simulink library "Lidar_WindReconstruction_16b"  (Simulink 8.8)
settings: Solver=VariableStepAuto  StartTime=0.0  StopTime=10.0  RelTol=1e-3
undefined symbols (not defined in the file): Atmosphere, CRM, LIDAR, SimConfig, WindReconstruction
libraries: simulink x1
settings Model: Creator=cava_da  LastModifiedBy=cava_da

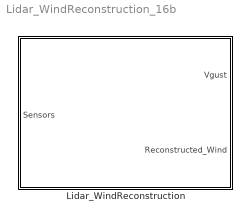
== system Lidar_WindReconstruction_16b ==
  Lidar_WindReconstruction : Subsystem

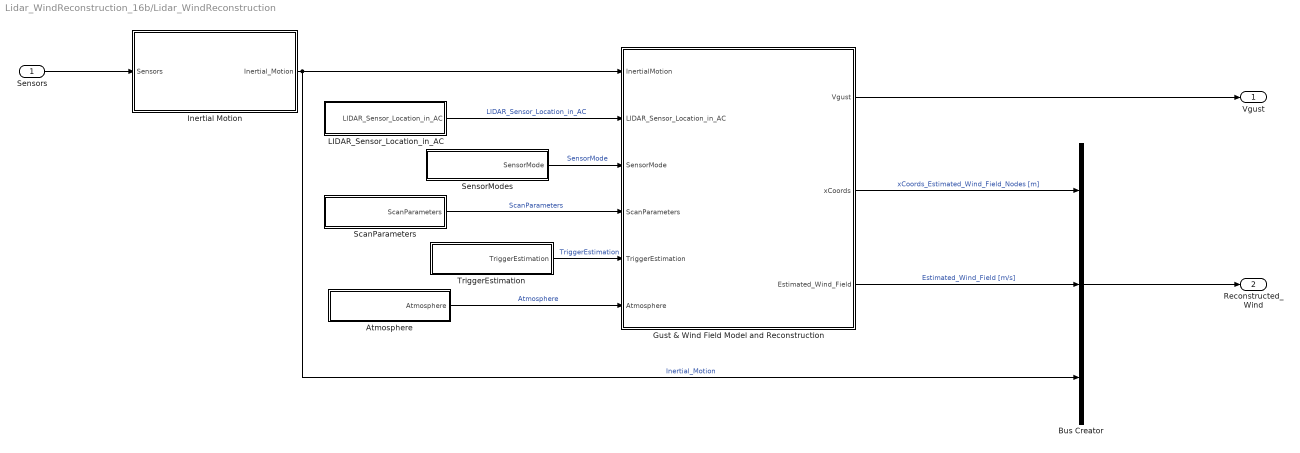
== system Lidar_WindReconstruction_16b/Lidar_WindReconstruction ==
  Sensors : Inport
  Atmosphere : Subsystem
  Bus Creator : BusCreator  Inputs=3
  Gust & Wind Field Model and Reconstruction : Subsystem
  Inertial Motion : Subsystem
  LIDAR_Sensor_Location_in_AC : Subsystem
  ScanParameters : Subsystem
  SensorModes : Subsystem
  TriggerEstimation : Subsystem
  Vgust : Outport
  Reconstructed_Wind : Outport  Port=2
  wires:
  Sensors/1 -> Inertial Motion/1(Sensors)
  LIDAR_Sensor_Location_in_AC/1(LIDAR_Sensor_Location_in_AC) -> Gust & Wind Field Model and Reconstruction/2(LIDAR_Sensor_Location_in_AC)  "LIDAR_Sensor_Location_in_AC"
  SensorModes/1(SensorMode) -> Gust & Wind Field Model and Reconstruction/3(SensorMode)  "SensorMode"
  ScanParameters/1(ScanParameters) -> Gust & Wind Field Model and Reconstruction/4(ScanParameters)  "ScanParameters"
  TriggerEstimation/1(TriggerEstimation) -> Gust & Wind Field Model and Reconstruction/5(TriggerEstimation)  "TriggerEstimation"
  Inertial Motion/1(Inertial_Motion) -> Bus Creator/3, Gust & Wind Field Model and Reconstruction/1(InertialMotion)  "Inertial_Motion"
  Gust & Wind Field Model and Reconstruction/2(xCoords) -> Bus Creator/1  "xCoords_Estimated_Wind_Field_Nodes [m]"
  Gust & Wind Field Model and Reconstruction/3(Estimated_Wind_Field) -> Bus Creator/2  "Estimated_Wind_Field [m/s]"
  Gust & Wind Field Model and Reconstruction/1(Vgust) -> Vgust/1
  Atmosphere/1(Atmosphere) -> Gust & Wind Field Model and Reconstruction/6(Atmosphere)  "Atmosphere"
  Bus Creator/1 -> Reconstructed_Wind/1

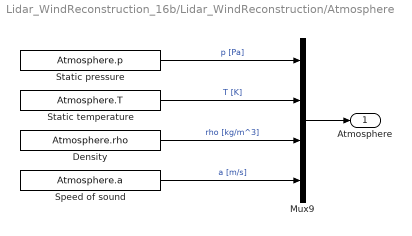
== system Lidar_WindReconstruction_16b/Lidar_WindReconstruction/Atmosphere ==
  Density : Constant  Value=Atmosphere.rho
  Mux9 : Mux
  Speed of sound : Constant  Value=Atmosphere.a
  Static pressure : Constant  Value=Atmosphere.p
  Static temperature : Constant  Value=Atmosphere.T
  Atmosphere : Outport
  wires:
  Mux9/1 -> Atmosphere/1
  Static pressure/1 -> Mux9/1  "p [Pa]"
  Static temperature/1 -> Mux9/2  "T [K]"
  Density/1 -> Mux9/3  "rho [kg/m^3]"
  Speed of sound/1 -> Mux9/4  "a [m/s]"

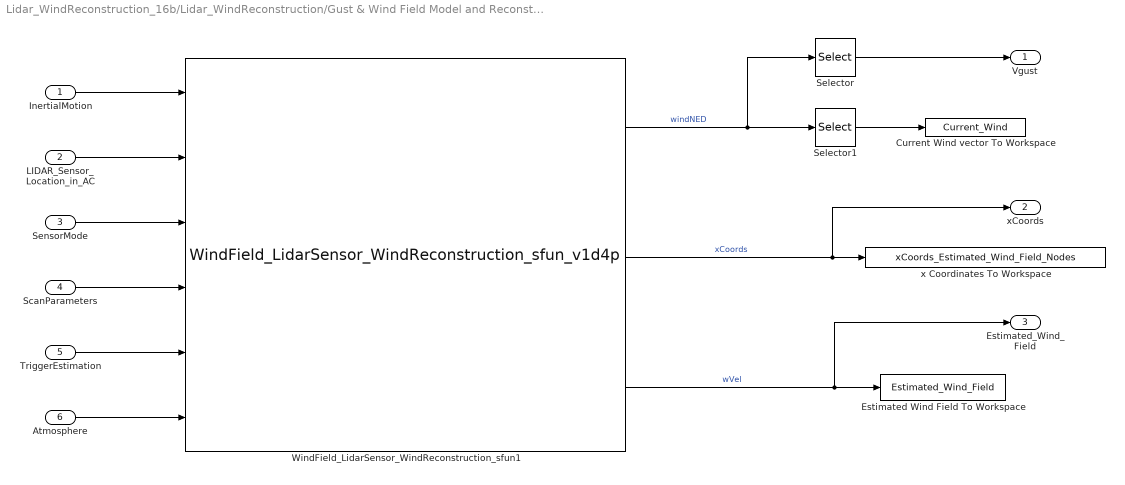
== system Lidar_WindReconstruction_16b/Lidar_WindReconstruction/Gust & Wind Field Model and Reconstruction ==
  InertialMotion : Inport
  LIDAR_Sensor_Location_in_AC : Inport  Port=2
  SensorMode : Inport  Port=3
  ScanParameters : Inport  Port=4
  TriggerEstimation : Inport  Port=5
  Atmosphere : Inport  Port=6
  Current Wind vector To Workspace : ToWorkspace  VariableName=Current_Wind  SaveFormat=Structure  SampleTime=-1
  Estimated Wind Field To Workspace : ToWorkspace  VariableName=Estimated_Wind_Field  SaveFormat=Structure With Time  SampleTime=0.1
      settings: Decimation=SimConfig.Logging.DecimationFactor
  Selector : Selector  IndexOptions=Index vector (dialog)  Indices=3  OutputSizes=1
  Selector1 : Selector  IndexOptions=Index vector (dialog)  Indices=1:3  OutputSizes=1
  WindField_LidarSensor_WindReconstruction_sfun1 : S-Function  FunctionName=WindField_LidarSensor_WindReconstruction_sfun_v1d4p  Parameters=Atmosphere,LIDAR,WindReconstruction  SFunctionDeploymentMode=off  EnableBusSupport=off  mask(Direct detection wind lidar and wind reconstruction (s-function)){}
      mask help:
      | This s-function incorporates the model of a direct detection Doppler wind lidar coupled with a wind reconstruction algorithm based on maximum likelihood estimation. It also serves as the interface between the included wind model and the encompassing aeroelastic aircraft model via the configurable wind output (output port 1).
      | The lidar model and the wind reconstruction algorithm are technically independent modules, but are implemented in the same s-function for performance reasons.
      |
      | Output port 1: wind output, configurable via the parameter Atmosphere.WindConfig
      | Output port 2: x-coordinates of the estimation nodes in geodetic frame and in meters
      | Output port 3: vertical wind speed at the estimation nodes in m/s
      |
      | Output ports 2 and 3 are only updated when a new estimation was triggered via input port 5.
      |
      | Detailed documentation is found under: https://github.com/dlr-ft-gla/GLA-Benchmark/wiki
      |
      |
      |
      | (c) Copyright 2021 DLR e. V.
      |
      | Institute of Flight Systems, 38108 Braunschweig, Germany.
      | Institute of Atmospheric Physics, 82234 Wessling, Germany.
      |
      | Authors:
      | Daniel Kiehn (daniel.kiehn@dlr.de)
      | Nicolas Fezans (nicolas.fezans@dlr.de)
      | Patrick Vrancken (patrick.vrancken@dlr.de)
      |
      | Block and underlying s-function released under CC-BY-ND 4.0 license.
      | https://creativecommons.org/licenses/by-nd/4.0/
      mask Help: For help, please refer to the online documentation of the CRM benchmark model: <a href="matlab: web('https://github.com/dlr-ft-gla/GLA-Benchmark/wiki')">https://github.com/dlr-ft-gla/GLA-Benchmark/wiki</a>.
      mask Display:
      | port_label('input', 1, 'Inertial motion');
      | port_label('input', 2, 'Sensor location in AC');
      | port_label('input', 3, 'Sensor mode');
      | port_label('input', 4, 'Scan parameters');
      | port_label('input', 5, 'Estimation trigger');
      | port_label('input', 6, 'Atmosphere');
      | 
      | port_label('output', 1, 'AC wind inputs');
      | port_label('output', 2, 'x coordinates');
      | port_label('output', 3, 'Estimated wind');
      | 
      | image(imread('DLR_Logo.jpg'),[180,10,81,68])
      | 
      | disp(['DIRECT DETECTION WIND LIDAR\n',...
      | '& WIND RECONSTRUCTION ALGORITHM\n\n\n\n',...
      | '(c) Copyright 2021 DLR e. V.\n\n',...
      | 'Institute of Flight Systems\n',...
      | 'Institute of Atmospheric Physics\n\n',...
      | 'Authors:\n',...
      | 'Daniel Kiehn (daniel.kiehn@dlr.de)\n',...
      | 'Nicolas Fezans (nicolas.fezans@dlr.de)\n',...
      | 'Patrick Vrancken (patrick.vrancken@dlr.de)\n\n\n',...
      | 'Block and underlying s-function\n',...
      | 'released under CC-BY-ND 4.0 license.'])
  x Coordinates To Workspace : ToWorkspace  VariableName=xCoords_Estimated_Wind_Field_Nodes  SaveFormat=Structure With Time  SampleTime=0.1
      settings: Decimation=SimConfig.Logging.DecimationFactor
  Vgust : Outport
  xCoords : Outport  Port=2
  Estimated_Wind_Field : Outport  Port=3
  wires:
  WindField_LidarSensor_WindReconstruction_sfun1/3 -> Estimated_Wind_Field/1, Estimated Wind Field To Workspace/1  "wVel"
  WindField_LidarSensor_WindReconstruction_sfun1/2 -> xCoords/1, x Coordinates To Workspace/1  "xCoords"
  WindField_LidarSensor_WindReconstruction_sfun1/1 -> Selector1/1, Selector/1  "windNED"
  InertialMotion/1 -> WindField_LidarSensor_WindReconstruction_sfun1/1
  LIDAR_Sensor_Location_in_AC/1 -> WindField_LidarSensor_WindReconstruction_sfun1/2
  SensorMode/1 -> WindField_LidarSensor_WindReconstruction_sfun1/3
  ScanParameters/1 -> WindField_LidarSensor_WindReconstruction_sfun1/4
  TriggerEstimation/1 -> WindField_LidarSensor_WindReconstruction_sfun1/5
  Selector/1 -> Vgust/1
  Atmosphere/1 -> WindField_LidarSensor_WindReconstruction_sfun1/6
  Selector1/1 -> Current Wind vector To Workspace/1

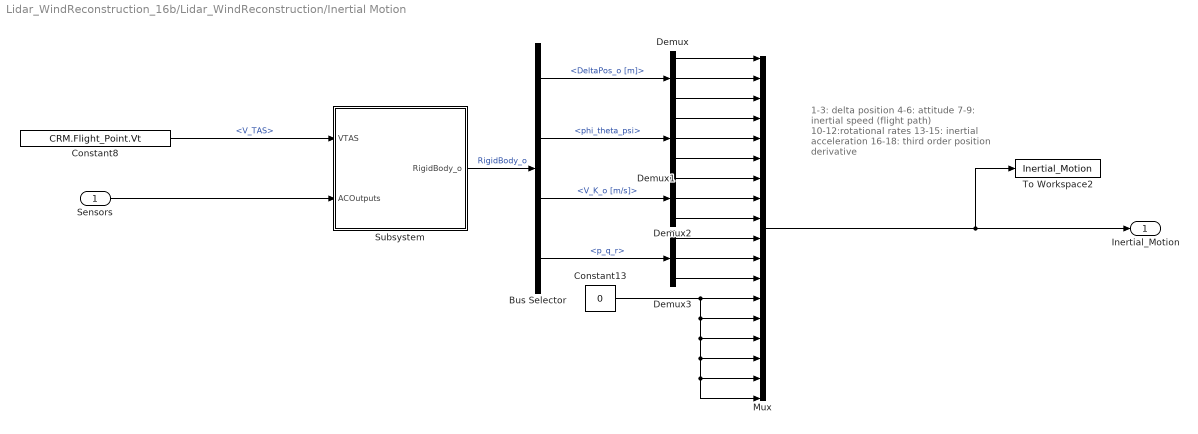
== system Lidar_WindReconstruction_16b/Lidar_WindReconstruction/Inertial Motion ==
  note: 1-3: delta position
      | 4-6: attitude
      | 7-9: inertial speed (flight path)
      | 10-12:rotational rates
      | 13-15: inertial acceleration
      | 16-18: third order position derivative
  Sensors : Inport
  Bus Selector : BusSelector  OutputSignals=DeltaPos_o [m],phi_theta_psi,V_K_o [m/s],p_q_r
  Constant13 : Constant  Value=0
  Constant8 : Constant  Value=CRM.Flight_Point.Vt
  Demux{,1..3} (4 alike) : Demux  Outputs=3
  Mux : Mux  Inputs=18
  Subsystem : Subsystem
  To Workspace2 : ToWorkspace  VariableName=Inertial_Motion  SaveFormat=Structure  SampleTime=-1
      settings: Decimation=SimConfig.Logging.DecimationFactor
  Inertial_Motion : Outport
  wires:
  Bus Selector/4 -> Demux3/1  "<p_q_r>"
  Bus Selector/1 -> Demux/1  "<DeltaPos_o [m]>"
  Bus Selector/2 -> Demux1/1  "<phi_theta_psi>"
  Bus Selector/3 -> Demux2/1  "<V_K_o [m/s]>"
  Demux/1 -> Mux/1
  Demux/2 -> Mux/2
  Demux/3 -> Mux/3
  Demux1/1 -> Mux/4
  Demux1/2 -> Mux/5
  Demux1/3 -> Mux/6
  Demux2/1 -> Mux/7
  Demux2/2 -> Mux/8
  Demux2/3 -> Mux/9
  Demux3/1 -> Mux/10
  Demux3/2 -> Mux/11
  Demux3/3 -> Mux/12
  Sensors/1 -> Subsystem/2(ACOutputs)
  Subsystem/1(RigidBody_o) -> Bus Selector/1  "RigidBody_o"
  Constant8/1 -> Subsystem/1(VTAS)  "<V_TAS>"
  Mux/1 -> Inertial_Motion/1, To Workspace2/1
  Constant13/1 -> Mux/17, Mux/18, Mux/16, Mux/15, Mux/14, Mux/13

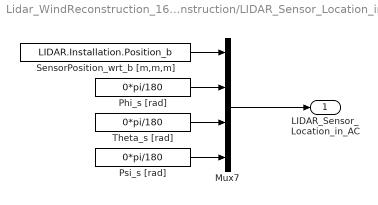
== system Lidar_WindReconstruction_16b/Lidar_WindReconstruction/LIDAR_Sensor_Location_in_AC ==
  Mux7 : Mux
  Phi_s [rad] : Constant  Value=0*pi/180
  Psi_s [rad] : Constant  Value=0*pi/180
  SensorPosition_wrt_b [m,m,m] : Constant  Value=LIDAR.Installation.Position_b
  Theta_s [rad] : Constant  Value=0*pi/180
  LIDAR_Sensor_Location_in_AC : Outport
  wires:
  SensorPosition_wrt_b [m,m,m]/1 -> Mux7/1
  Phi_s [rad]/1 -> Mux7/2
  Theta_s [rad]/1 -> Mux7/3
  Psi_s [rad]/1 -> Mux7/4
  Mux7/1 -> LIDAR_Sensor_Location_in_AC/1

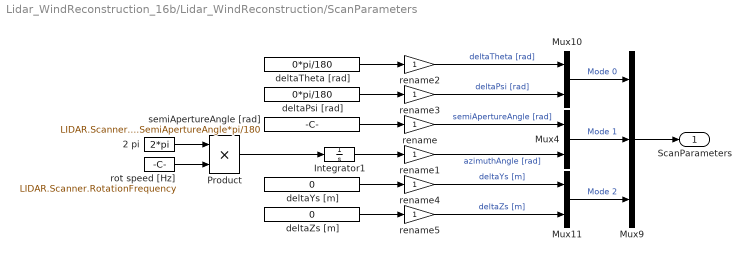
== system Lidar_WindReconstruction_16b/Lidar_WindReconstruction/ScanParameters ==
  2 pi : Constant  Value=2*pi
  Integrator1 : Integrator
  Mux10 : Mux  Inputs=2
  Mux11 : Mux  Inputs=2
  Mux4 : Mux  Inputs=2
  Mux9 : Mux  Inputs=3
  Product : Product  RndMeth=Zero
  deltaPsi [rad] : Constant  Value=0*pi/180  OutDataTypeStr=double
  deltaTheta [rad] : Constant  Value=0*pi/180  OutDataTypeStr=double
  deltaYs [m] : Constant  Value=0  OutDataTypeStr=double
  deltaZs [m] : Constant  Value=0  OutDataTypeStr=double
  rename{,1..5} (6 alike) : Gain
  rot speed [Hz] : Constant  Value=LIDAR.Scanner.RotationFrequency
  semiApertureAngle [rad] : Constant  Value=LIDAR.Scanner.SemiApertureAngle*pi/180  OutDataTypeStr=double
  ScanParameters : Outport
  wires:
  rename3/1 -> Mux10/2  "deltaPsi [rad]"
  rename2/1 -> Mux10/1  "deltaTheta [rad]"
  Mux10/1 -> Mux9/1  "Mode 0"
  rename1/1 -> Mux4/2  "azimuthAngle [rad]"
  rename/1 -> Mux4/1  "semiApertureAngle [rad]"
  rename5/1 -> Mux11/2  "deltaZs [m]"
  rename4/1 -> Mux11/1  "deltaYs [m]"
  Mux4/1 -> Mux9/2  "Mode 1"
  Mux11/1 -> Mux9/3  "Mode 2"
  deltaPsi [rad]/1 -> rename3/1
  deltaTheta [rad]/1 -> rename2/1
  deltaYs [m]/1 -> rename4/1
  deltaZs [m]/1 -> rename5/1
  semiApertureAngle [rad]/1 -> rename/1
  2 pi/1 -> Product/1
  Product/1 -> Integrator1/1
  rot speed [Hz]/1 -> Product/2
  Integrator1/1 -> rename1/1
  Mux9/1 -> ScanParameters/1

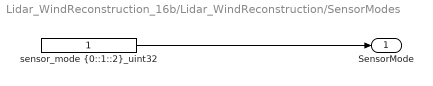
== system Lidar_WindReconstruction_16b/Lidar_WindReconstruction/SensorModes ==
  "sensor_mode {0::1::2}_uint32" : Constant  OutDataTypeStr=uint32
  SensorMode : Outport
  wires:
  "sensor_mode {0::1::2}_uint32"/1 -> SensorMode/1

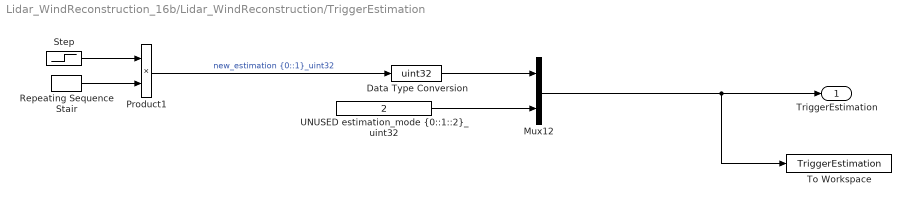
== system Lidar_WindReconstruction_16b/Lidar_WindReconstruction/TriggerEstimation ==
  Data Type Conversion : DataTypeConversion  OutDataTypeStr=uint32
  Mux12 : Mux  Inputs=2
  Product1 : Product  RndMeth=Zero
  Repeating Sequence Stair : simulink/Sources/Repeating Sequence Stair  OutValues=[1 zeros(1,(1/(10*SimConfig.SampleTime))-1)].'  tsamp=-1  OutMin=[]  OutMax=[]  OutDataTypeStr=float('double')  OutputDataTypeScalingMode=Specify via dialog  OutDataType=float('double')  ConRadixGroup=Best Precision: Vector-wise  OutScaling=2^-12
  Step : Step  Time=WindReconstruction.StartEstimationTime  SampleTime=0
  To Workspace : ToWorkspace  VariableName=TriggerEstimation  SaveFormat=Structure  SampleTime=-1
  "UNUSED estimation_mode {0::1::2}_uint32" : Constant  Value=2  OutDataTypeStr=uint32
  TriggerEstimation : Outport
  wires:
  Product1/1 -> Data Type Conversion/1  "new_estimation {0::1}_uint32"
  "UNUSED estimation_mode {0::1::2}_uint32"/1 -> Mux12/2
  Data Type Conversion/1 -> Mux12/1
  Repeating Sequence Stair/1 -> Product1/2
  Step/1 -> Product1/1
  Mux12/1 -> TriggerEstimation/1, To Workspace/1

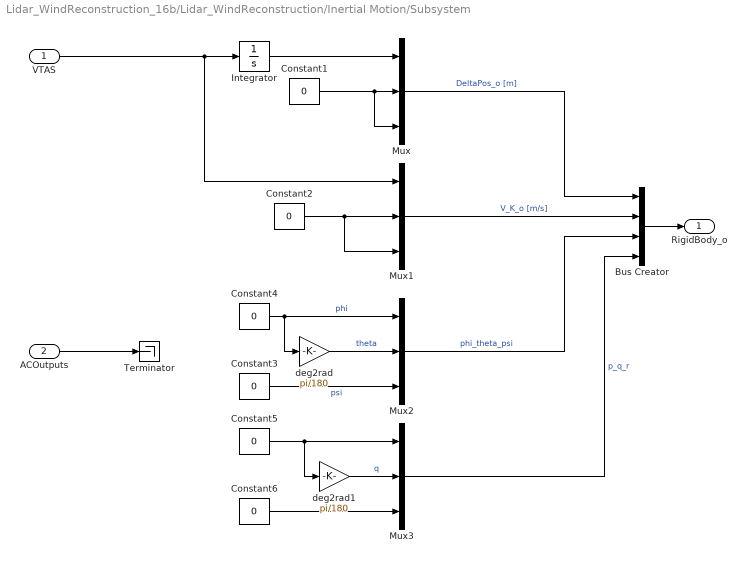
== system Lidar_WindReconstruction_16b/Lidar_WindReconstruction/Inertial Motion/Subsystem ==
  VTAS : Inport
  ACOutputs : Inport  Port=2
  Bus Creator : BusCreator  Inputs=4
  Constant{1..6} (6 alike) : Constant  Value=0
  Integrator : Integrator
  Mux{,1..3} (4 alike) : Mux  Inputs=3
  Terminator : Terminator
  deg2rad : Gain  Gain=pi/180
  deg2rad1 : Gain  Gain=pi/180
  RigidBody_o : Outport
  wires:
  Constant1/1 -> Mux/2, Mux/3
  Integrator/1 -> Mux/1
  Mux/1 -> Bus Creator/1  "DeltaPos_o [m]"
  Bus Creator/1 -> RigidBody_o/1
  Mux1/1 -> Bus Creator/2  "V_K_o [m/s]"
  Constant2/1 -> Mux1/2, Mux1/3
  Mux2/1 -> Bus Creator/3  "phi_theta_psi"
  Constant4/1 -> Mux2/1, deg2rad/1  "phi"
  deg2rad/1 -> Mux2/2  "theta"
  Constant3/1 -> Mux2/3  "psi"
  Mux3/1 -> Bus Creator/4  "p_q_r"
  deg2rad1/1 -> Mux3/2  "q"
  Constant5/1 -> Mux3/1, deg2rad1/1
  Constant6/1 -> Mux3/3
  VTAS/1 -> Mux1/1, Integrator/1
  ACOutputs/1 -> Terminator/1
